simulink model "PWMGenerator"  (R2017a)
settings: Solver=VariableStepAuto  StartTime=0.0  StopTime=10.0  RelTol=1e-3
libraries: hdlsllib x15, simulink x5
settings Model: Creator=zhao.yi4  LastModifiedBy=zhao.yi4
settings OptimizationCC: BlockReduction=off  ConditionallyExecuteInputs=off  DefaultParameterBehavior=Inlined
settings DebuggingCC: AlgebraicLoopMsg=error
settings HardwareCC: ProdBitPerPointer=32  ProdBitPerSizeT=32  ProdBitPerPtrDiffT=32  ProdLargestAtomicFloat=None  ProdIntDivRoundTo=Undefined  ProdEndianess=Unspecified  ProdWordSize=32  ProdHWDeviceType=ASIC/FPGA->ASIC/FPGA  ProdEqTarget=off

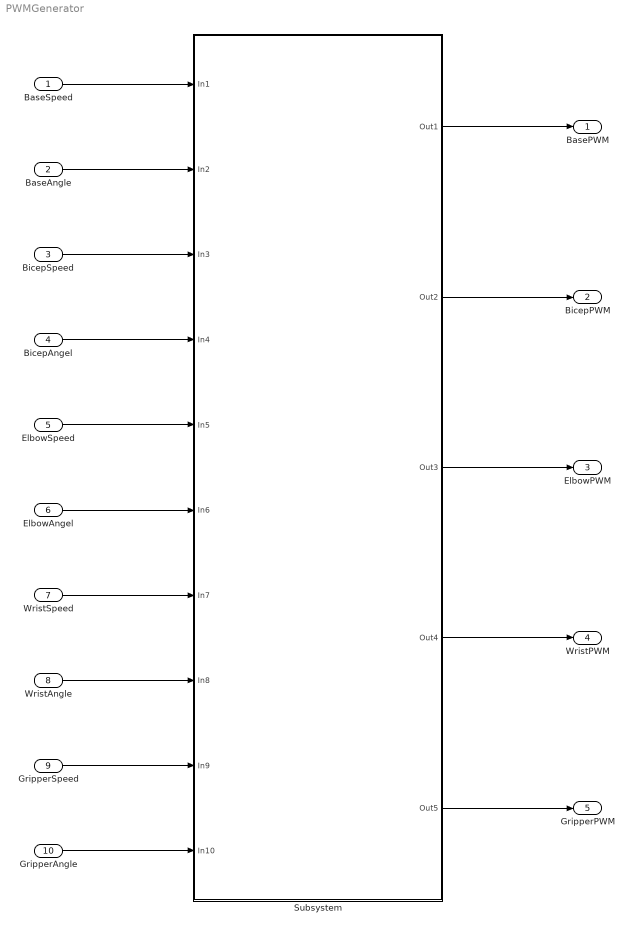
== system PWMGenerator ==
  BaseSpeed : Inport  OutDataTypeStr=uint8  SampleTime=1
  BaseAngle : Inport  Port=2  OutDataTypeStr=uint8  SampleTime=1
  BicepSpeed : Inport  Port=3  OutDataTypeStr=uint8  SampleTime=1
  BicepAngel : Inport  Port=4  OutDataTypeStr=uint8  SampleTime=1
  ElbowSpeed : Inport  Port=5  OutDataTypeStr=uint8  SampleTime=1
  ElbowAngel : Inport  Port=6  OutDataTypeStr=uint8  SampleTime=1
  WristSpeed : Inport  Port=7  OutDataTypeStr=uint8  SampleTime=1
  WristAngle : Inport  Port=8  OutDataTypeStr=uint8  SampleTime=1
  GripperSpeed : Inport  Port=9  OutDataTypeStr=uint8  SampleTime=1
  GripperAngle : Inport  Port=10  OutDataTypeStr=uint8  SampleTime=1
  Subsystem : Subsystem
  "BasePWM " : Outport  SampleTime=1
  "BicepPWM " : Outport  Port=2  SampleTime=1
  "ElbowPWM " : Outport  Port=3  SampleTime=1
  "WristPWM " : Outport  Port=4  SampleTime=1
  "GripperPWM " : Outport  Port=5  SampleTime=1
  wires:
  BaseSpeed/1 -> Subsystem/1(In1)
  BaseAngle/1 -> Subsystem/2(In2)
  BicepSpeed/1 -> Subsystem/3(In3)
  BicepAngel/1 -> Subsystem/4(In4)
  ElbowSpeed/1 -> Subsystem/5(In5)
  ElbowAngel/1 -> Subsystem/6(In6)
  WristSpeed/1 -> Subsystem/7(In7)
  WristAngle/1 -> Subsystem/8(In8)
  GripperSpeed/1 -> Subsystem/9(In9)
  GripperAngle/1 -> Subsystem/10(In10)
  Subsystem/1(Out1) -> "BasePWM "/1
  Subsystem/2(Out2) -> "BicepPWM "/1
  Subsystem/3(Out3) -> "ElbowPWM "/1
  Subsystem/4(Out4) -> "WristPWM "/1
  Subsystem/5(Out5) -> "GripperPWM "/1

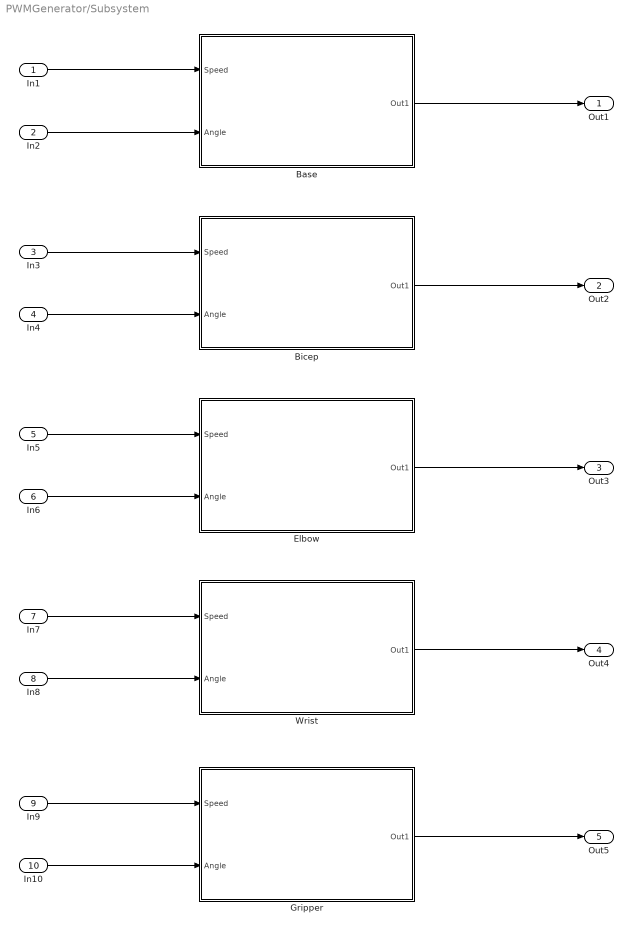
== system PWMGenerator/Subsystem ==
  In1 : Inport
  In2 : Inport  Port=2
  In3 : Inport  Port=3
  In4 : Inport  Port=4
  In5 : Inport  Port=5
  In6 : Inport  Port=6
  In7 : Inport  Port=7
  In8 : Inport  Port=8
  In9 : Inport  Port=9
  In10 : Inport  Port=10
  Base : Subsystem
  Bicep : Subsystem
  Elbow : Subsystem
  Gripper : Subsystem
  Wrist : Subsystem
  Out1 : Outport
  Out2 : Outport  Port=2
  Out3 : Outport  Port=3
  Out4 : Outport  Port=4
  Out5 : Outport  Port=5
  wires:
  Bicep/1(Out1) -> Out2/1
  In3/1 -> Bicep/1("Speed ")
  In4/1 -> Bicep/2(Angle)
  In1/1 -> Base/1("Speed ")
  In2/1 -> Base/2(Angle)
  Base/1(Out1) -> Out1/1
  In7/1 -> Wrist/1("Speed ")
  Wrist/1(Out1) -> Out4/1
  In8/1 -> Wrist/2(Angle)
  Elbow/1(Out1) -> Out3/1
  In6/1 -> Elbow/2(Angle)
  In5/1 -> Elbow/1("Speed ")
  Gripper/1(Out1) -> Out5/1
  In9/1 -> Gripper/1("Speed ")
  In10/1 -> Gripper/2(Angle)

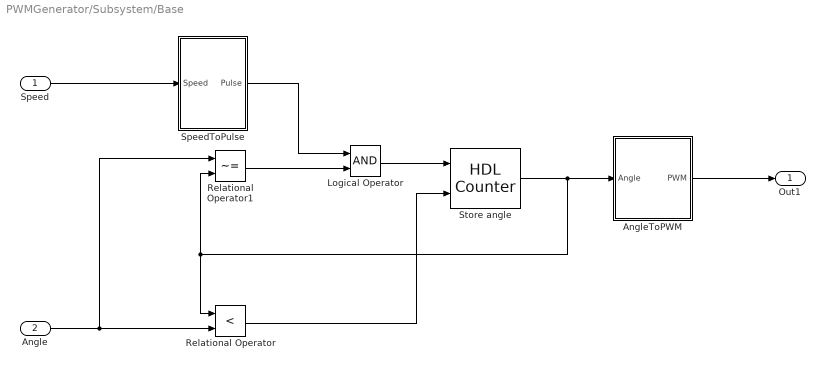
== system PWMGenerator/Subsystem/Base ==
  "Speed " : Inport  SampleTime=1
  Angle : Inport  Port=2  SampleTime=1
  "AngleToPWM " : Subsystem
  Logical Operator : Logic  AllPortsSameDT=off  OutDataTypeStr=boolean
  Relational Operator : RelationalOperator  Operator=<  OutDataTypeStr=boolean  RndMeth=Simplest
  Relational Operator1 : RelationalOperator  Operator=~=  OutDataTypeStr=boolean  RndMeth=Simplest
  SpeedToPulse : Subsystem
  Store angle : hdlsllib/HDL Operations/HDL Counter  CountType=Count limited  CountInit=90  CountStep=1  CountMax=185  CountFromType=Initial value  CountFrom=90  CountResetPort=off  CountLoadPort=off  CountEnbPort=on  CountDirPort=on  CountDataType=Unsigned  CountWordLen=8  CountFracLen=0  CountSampTime=1
      settings: SourceProductName=HDL Coder  SourceProductBaseCode=HD
  Out1 : Outport  SampleTime=1
  wires:
  "AngleToPWM "/1("PWM ") -> Out1/1
  Logical Operator/1 -> Store angle/1
  Store angle/1 -> Relational Operator1/2, Relational Operator/1, "AngleToPWM "/1(Angle)
  Relational Operator/1 -> Store angle/2
  Angle/1 -> Relational Operator1/1, Relational Operator/2
  SpeedToPulse/1("Pulse ") -> Logical Operator/1
  "Speed "/1 -> SpeedToPulse/1(Speed)
  Relational Operator1/1 -> Logical Operator/2

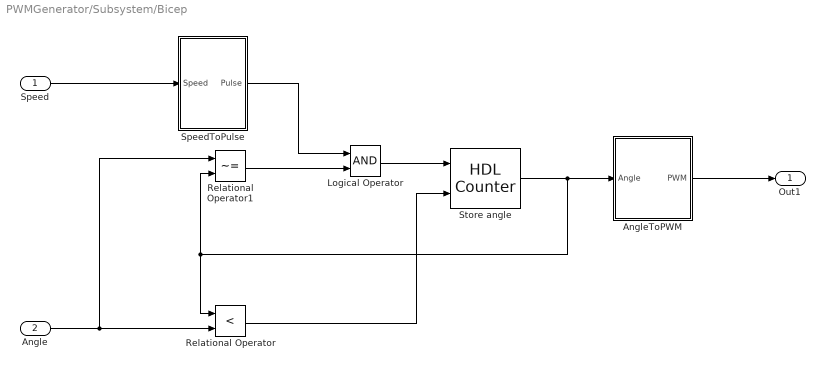
== system PWMGenerator/Subsystem/Bicep ==
  "Speed " : Inport  SampleTime=1
  Angle : Inport  Port=2  SampleTime=1
  "AngleToPWM " : Subsystem
  Logical Operator : Logic  AllPortsSameDT=off  OutDataTypeStr=boolean
  Relational Operator : RelationalOperator  Operator=<  OutDataTypeStr=boolean  RndMeth=Simplest
  Relational Operator1 : RelationalOperator  Operator=~=  OutDataTypeStr=boolean  RndMeth=Simplest
  SpeedToPulse : Subsystem
  Store angle : hdlsllib/HDL Operations/HDL Counter  CountType=Count limited  CountInit=90  CountStep=1  CountMax=185  CountFromType=Initial value  CountFrom=90  CountResetPort=off  CountLoadPort=off  CountEnbPort=on  CountDirPort=on  CountDataType=Unsigned  CountWordLen=8  CountFracLen=0  CountSampTime=1
      settings: SourceProductName=HDL Coder  SourceProductBaseCode=HD
  Out1 : Outport  SampleTime=1
  wires:
  "AngleToPWM "/1("PWM ") -> Out1/1
  Logical Operator/1 -> Store angle/1
  Store angle/1 -> Relational Operator1/2, Relational Operator/1, "AngleToPWM "/1(Angle)
  Relational Operator/1 -> Store angle/2
  Angle/1 -> Relational Operator1/1, Relational Operator/2
  SpeedToPulse/1("Pulse ") -> Logical Operator/1
  "Speed "/1 -> SpeedToPulse/1(Speed)
  Relational Operator1/1 -> Logical Operator/2

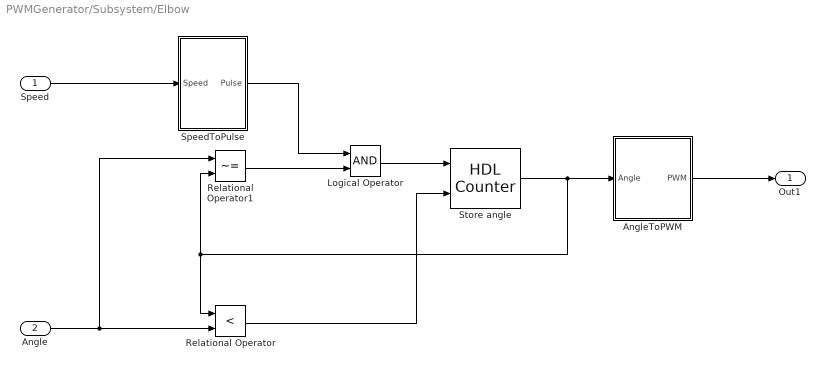
== system PWMGenerator/Subsystem/Elbow ==
  "Speed " : Inport  SampleTime=1
  Angle : Inport  Port=2  SampleTime=1
  "AngleToPWM " : Subsystem
  Logical Operator : Logic  AllPortsSameDT=off  OutDataTypeStr=boolean
  Relational Operator : RelationalOperator  Operator=<  OutDataTypeStr=boolean  RndMeth=Simplest
  Relational Operator1 : RelationalOperator  Operator=~=  OutDataTypeStr=boolean  RndMeth=Simplest
  SpeedToPulse : Subsystem
  Store angle : hdlsllib/HDL Operations/HDL Counter  CountType=Count limited  CountInit=90  CountStep=1  CountMax=185  CountFromType=Initial value  CountFrom=90  CountResetPort=off  CountLoadPort=off  CountEnbPort=on  CountDirPort=on  CountDataType=Unsigned  CountWordLen=8  CountFracLen=0  CountSampTime=1
      settings: SourceProductName=HDL Coder  SourceProductBaseCode=HD
  Out1 : Outport  SampleTime=1
  wires:
  "AngleToPWM "/1("PWM ") -> Out1/1
  Logical Operator/1 -> Store angle/1
  Store angle/1 -> Relational Operator1/2, Relational Operator/1, "AngleToPWM "/1(Angle)
  Relational Operator/1 -> Store angle/2
  Angle/1 -> Relational Operator1/1, Relational Operator/2
  SpeedToPulse/1("Pulse ") -> Logical Operator/1
  "Speed "/1 -> SpeedToPulse/1(Speed)
  Relational Operator1/1 -> Logical Operator/2

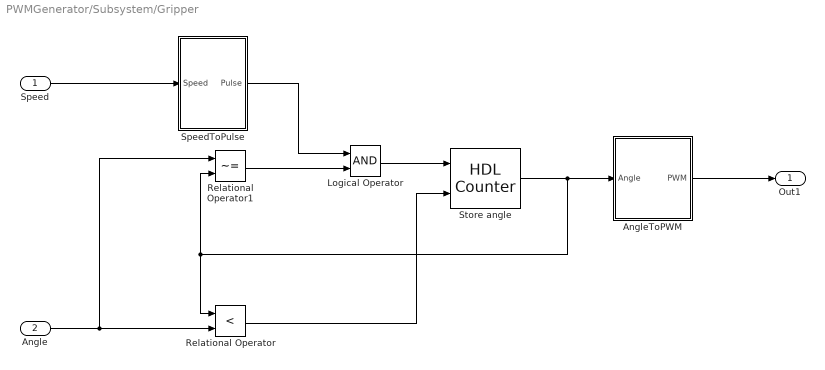
== system PWMGenerator/Subsystem/Gripper ==
  "Speed " : Inport  SampleTime=1
  Angle : Inport  Port=2  SampleTime=1
  "AngleToPWM " : Subsystem
  Logical Operator : Logic  AllPortsSameDT=off  OutDataTypeStr=boolean
  Relational Operator : RelationalOperator  Operator=<  OutDataTypeStr=boolean  RndMeth=Simplest
  Relational Operator1 : RelationalOperator  Operator=~=  OutDataTypeStr=boolean  RndMeth=Simplest
  SpeedToPulse : Subsystem
  Store angle : hdlsllib/HDL Operations/HDL Counter  CountType=Count limited  CountInit=90  CountStep=1  CountMax=185  CountFromType=Initial value  CountFrom=90  CountResetPort=off  CountLoadPort=off  CountEnbPort=on  CountDirPort=on  CountDataType=Unsigned  CountWordLen=8  CountFracLen=0  CountSampTime=1
      settings: SourceProductName=HDL Coder  SourceProductBaseCode=HD
  Out1 : Outport  SampleTime=1
  wires:
  "AngleToPWM "/1("PWM ") -> Out1/1
  Logical Operator/1 -> Store angle/1
  Store angle/1 -> Relational Operator1/2, Relational Operator/1, "AngleToPWM "/1(Angle)
  Relational Operator/1 -> Store angle/2
  Angle/1 -> Relational Operator1/1, Relational Operator/2
  SpeedToPulse/1("Pulse ") -> Logical Operator/1
  "Speed "/1 -> SpeedToPulse/1(Speed)
  Relational Operator1/1 -> Logical Operator/2

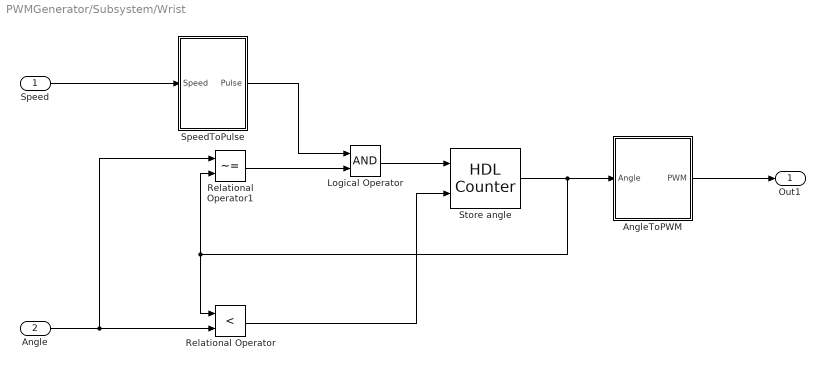
== system PWMGenerator/Subsystem/Wrist ==
  "Speed " : Inport  SampleTime=1
  Angle : Inport  Port=2  SampleTime=1
  "AngleToPWM " : Subsystem
  Logical Operator : Logic  AllPortsSameDT=off  OutDataTypeStr=boolean
  Relational Operator : RelationalOperator  Operator=<  OutDataTypeStr=boolean  RndMeth=Simplest
  Relational Operator1 : RelationalOperator  Operator=~=  OutDataTypeStr=boolean  RndMeth=Simplest
  SpeedToPulse : Subsystem
  Store angle : hdlsllib/HDL Operations/HDL Counter  CountType=Count limited  CountInit=90  CountStep=1  CountMax=185  CountFromType=Initial value  CountFrom=90  CountResetPort=off  CountLoadPort=off  CountEnbPort=on  CountDirPort=on  CountDataType=Unsigned  CountWordLen=8  CountFracLen=0  CountSampTime=1
      settings: SourceProductName=HDL Coder  SourceProductBaseCode=HD
  Out1 : Outport  SampleTime=1
  wires:
  "AngleToPWM "/1("PWM ") -> Out1/1
  Logical Operator/1 -> Store angle/1
  Store angle/1 -> Relational Operator1/2, Relational Operator/1, "AngleToPWM "/1(Angle)
  Relational Operator/1 -> Store angle/2
  Angle/1 -> Relational Operator1/1, Relational Operator/2
  SpeedToPulse/1("Pulse ") -> Logical Operator/1
  "Speed "/1 -> SpeedToPulse/1(Speed)
  Relational Operator1/1 -> Logical Operator/2

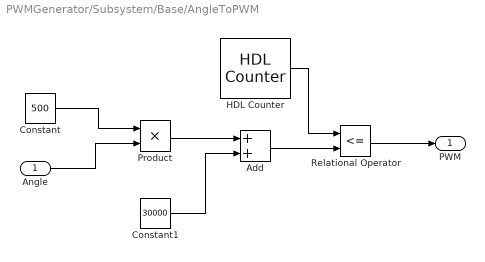
== system PWMGenerator/Subsystem/Base/AngleToPWM  ==
  Angle : Inport  OutDataTypeStr=uint8  SampleTime=1
  Add : Sum  AccumDataTypeStr=uint32  OutDataTypeStr=uint32
  Constant : Constant  Value=500  OutDataTypeStr=uint32  SampleTime=1
  Constant1 : Constant  Value=30000  OutDataTypeStr=uint32  SampleTime=1
  HDL Counter : hdlsllib/HDL Operations/HDL Counter  CountType=Count limited  CountInit=0  CountStep=1  CountMax=1000000  CountFromType=Initial value  CountFrom=0  CountResetPort=off  CountLoadPort=off  CountEnbPort=off  CountDirPort=off  CountDataType=Unsigned  CountWordLen=32  CountFracLen=0  CountSampTime=1
      settings: SourceProductName=HDL Coder  SourceProductBaseCode=HD
  Product : Product  OutDataTypeStr=uint32
  Relational Operator : RelationalOperator  Operator=<=  OutDataTypeStr=boolean  RndMeth=Simplest
  "PWM " : Outport  SampleTime=1
  wires:
  Product/1 -> Add/1
  Angle/1 -> Product/2
  Constant/1 -> Product/1
  HDL Counter/1 -> Relational Operator/1
  Relational Operator/1 -> "PWM "/1
  Add/1 -> Relational Operator/2
  Constant1/1 -> Add/2

== system PWMGenerator/Subsystem/Base/SpeedToPulse ==
  Speed : Inport  OutDataTypeStr=uint8  SampleTime=1
  Compare To Constant : simulink/Logic and Bit Operations/Compare To Constant  relop===  const=0  OutDataTypeStr=boolean
  Cycles in a second : Constant  Value=50000000  OutDataTypeStr=uint32  SampleTime=1
  Divide : Product  Inputs=*/  SaturateOnIntegerOverflow=on  RndMeth=Zero
  HDL Counter : hdlsllib/HDL Operations/HDL Counter  CountType=Free running  CountInit=0  CountStep=1  CountMax=25  CountFromType=Initial value  CountFrom=0  CountResetPort=on  CountLoadPort=off  CountEnbPort=off  CountDirPort=off  CountDataType=Unsigned  CountWordLen=32  CountFracLen=0  CountSampTime=1
      settings: SourceProductName=HDL Coder  SourceProductBaseCode=HD
  Relational Operator : RelationalOperator  Operator=>  OutDataTypeStr=boolean  RndMeth=Simplest
  "Pulse " : Outport  SampleTime=1
  wires:
  HDL Counter/1 -> Relational Operator/1, Compare To Constant/1
  Speed/1 -> Divide/2
  Relational Operator/1 -> HDL Counter/1
  Cycles in a second/1 -> Divide/1
  Divide/1 -> Relational Operator/2
  Compare To Constant/1 -> "Pulse "/1

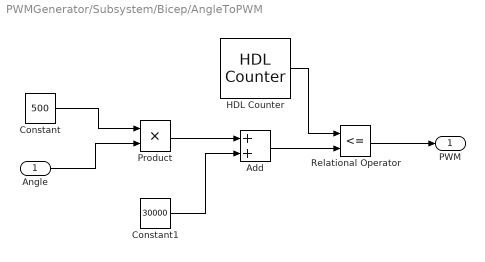
== system PWMGenerator/Subsystem/Bicep/AngleToPWM  ==
  Angle : Inport  OutDataTypeStr=uint8  SampleTime=1
  Add : Sum  AccumDataTypeStr=uint32  OutDataTypeStr=uint32
  Constant : Constant  Value=500  OutDataTypeStr=uint32  SampleTime=1
  Constant1 : Constant  Value=30000  OutDataTypeStr=uint32  SampleTime=1
  HDL Counter : hdlsllib/HDL Operations/HDL Counter  CountType=Count limited  CountInit=0  CountStep=1  CountMax=1000000  CountFromType=Initial value  CountFrom=0  CountResetPort=off  CountLoadPort=off  CountEnbPort=off  CountDirPort=off  CountDataType=Unsigned  CountWordLen=32  CountFracLen=0  CountSampTime=1
      settings: SourceProductName=HDL Coder  SourceProductBaseCode=HD
  Product : Product  OutDataTypeStr=uint32
  Relational Operator : RelationalOperator  Operator=<=  OutDataTypeStr=boolean  RndMeth=Simplest
  "PWM " : Outport  SampleTime=1
  wires:
  Product/1 -> Add/1
  Angle/1 -> Product/2
  Constant/1 -> Product/1
  HDL Counter/1 -> Relational Operator/1
  Relational Operator/1 -> "PWM "/1
  Add/1 -> Relational Operator/2
  Constant1/1 -> Add/2

== system PWMGenerator/Subsystem/Bicep/SpeedToPulse ==
  Speed : Inport  OutDataTypeStr=uint8  SampleTime=1
  Compare To Constant : simulink/Logic and Bit Operations/Compare To Constant  relop===  const=0  OutDataTypeStr=boolean
  Cycles in a second : Constant  Value=50000000  OutDataTypeStr=uint32  SampleTime=1
  Divide : Product  Inputs=*/  SaturateOnIntegerOverflow=on  RndMeth=Zero
  HDL Counter : hdlsllib/HDL Operations/HDL Counter  CountType=Free running  CountInit=0  CountStep=1  CountMax=25  CountFromType=Initial value  CountFrom=0  CountResetPort=on  CountLoadPort=off  CountEnbPort=off  CountDirPort=off  CountDataType=Unsigned  CountWordLen=32  CountFracLen=0  CountSampTime=1
      settings: SourceProductName=HDL Coder  SourceProductBaseCode=HD
  Relational Operator : RelationalOperator  Operator=>  OutDataTypeStr=boolean  RndMeth=Simplest
  "Pulse " : Outport  SampleTime=1
  wires:
  HDL Counter/1 -> Relational Operator/1, Compare To Constant/1
  Speed/1 -> Divide/2
  Relational Operator/1 -> HDL Counter/1
  Cycles in a second/1 -> Divide/1
  Divide/1 -> Relational Operator/2
  Compare To Constant/1 -> "Pulse "/1

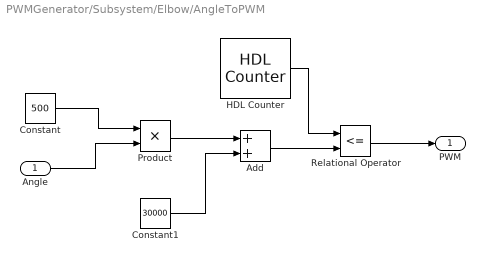
== system PWMGenerator/Subsystem/Elbow/AngleToPWM  ==
  Angle : Inport  OutDataTypeStr=uint8  SampleTime=1
  Add : Sum  AccumDataTypeStr=uint32  OutDataTypeStr=uint32
  Constant : Constant  Value=500  OutDataTypeStr=uint32  SampleTime=1
  Constant1 : Constant  Value=30000  OutDataTypeStr=uint32  SampleTime=1
  HDL Counter : hdlsllib/HDL Operations/HDL Counter  CountType=Count limited  CountInit=0  CountStep=1  CountMax=1000000  CountFromType=Initial value  CountFrom=0  CountResetPort=off  CountLoadPort=off  CountEnbPort=off  CountDirPort=off  CountDataType=Unsigned  CountWordLen=32  CountFracLen=0  CountSampTime=1
      settings: SourceProductName=HDL Coder  SourceProductBaseCode=HD
  Product : Product  OutDataTypeStr=uint32
  Relational Operator : RelationalOperator  Operator=<=  OutDataTypeStr=boolean  RndMeth=Simplest
  "PWM " : Outport  SampleTime=1
  wires:
  Product/1 -> Add/1
  Angle/1 -> Product/2
  Constant/1 -> Product/1
  HDL Counter/1 -> Relational Operator/1
  Relational Operator/1 -> "PWM "/1
  Add/1 -> Relational Operator/2
  Constant1/1 -> Add/2

== system PWMGenerator/Subsystem/Elbow/SpeedToPulse ==
  Speed : Inport  OutDataTypeStr=uint8  SampleTime=1
  Compare To Constant : simulink/Logic and Bit Operations/Compare To Constant  relop===  const=0  OutDataTypeStr=boolean
  Cycles in a second : Constant  Value=50000000  OutDataTypeStr=uint32  SampleTime=1
  Divide : Product  Inputs=*/  SaturateOnIntegerOverflow=on  RndMeth=Zero
  HDL Counter : hdlsllib/HDL Operations/HDL Counter  CountType=Free running  CountInit=0  CountStep=1  CountMax=25  CountFromType=Initial value  CountFrom=0  CountResetPort=on  CountLoadPort=off  CountEnbPort=off  CountDirPort=off  CountDataType=Unsigned  CountWordLen=32  CountFracLen=0  CountSampTime=1
      settings: SourceProductName=HDL Coder  SourceProductBaseCode=HD
  Relational Operator : RelationalOperator  Operator=>  OutDataTypeStr=boolean  RndMeth=Simplest
  "Pulse " : Outport  SampleTime=1
  wires:
  HDL Counter/1 -> Relational Operator/1, Compare To Constant/1
  Speed/1 -> Divide/2
  Relational Operator/1 -> HDL Counter/1
  Cycles in a second/1 -> Divide/1
  Divide/1 -> Relational Operator/2
  Compare To Constant/1 -> "Pulse "/1

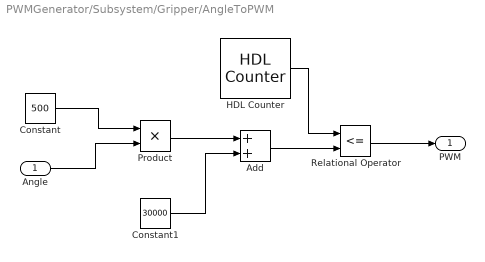
== system PWMGenerator/Subsystem/Gripper/AngleToPWM  ==
  Angle : Inport  OutDataTypeStr=uint8  SampleTime=1
  Add : Sum  AccumDataTypeStr=uint32  OutDataTypeStr=uint32
  Constant : Constant  Value=500  OutDataTypeStr=uint32  SampleTime=1
  Constant1 : Constant  Value=30000  OutDataTypeStr=uint32  SampleTime=1
  HDL Counter : hdlsllib/HDL Operations/HDL Counter  CountType=Count limited  CountInit=0  CountStep=1  CountMax=1000000  CountFromType=Initial value  CountFrom=0  CountResetPort=off  CountLoadPort=off  CountEnbPort=off  CountDirPort=off  CountDataType=Unsigned  CountWordLen=32  CountFracLen=0  CountSampTime=1
      settings: SourceProductName=HDL Coder  SourceProductBaseCode=HD
  Product : Product  OutDataTypeStr=uint32
  Relational Operator : RelationalOperator  Operator=<=  OutDataTypeStr=boolean  RndMeth=Simplest
  "PWM " : Outport  SampleTime=1
  wires:
  Product/1 -> Add/1
  Angle/1 -> Product/2
  Constant/1 -> Product/1
  HDL Counter/1 -> Relational Operator/1
  Relational Operator/1 -> "PWM "/1
  Add/1 -> Relational Operator/2
  Constant1/1 -> Add/2

== system PWMGenerator/Subsystem/Gripper/SpeedToPulse ==
  Speed : Inport  OutDataTypeStr=uint8  SampleTime=1
  Compare To Constant : simulink/Logic and Bit Operations/Compare To Constant  relop===  const=0  OutDataTypeStr=boolean
  Cycles in a second : Constant  Value=50000000  OutDataTypeStr=uint32  SampleTime=1
  Divide : Product  Inputs=*/  SaturateOnIntegerOverflow=on  RndMeth=Zero
  HDL Counter : hdlsllib/HDL Operations/HDL Counter  CountType=Free running  CountInit=0  CountStep=1  CountMax=25  CountFromType=Initial value  CountFrom=0  CountResetPort=on  CountLoadPort=off  CountEnbPort=off  CountDirPort=off  CountDataType=Unsigned  CountWordLen=32  CountFracLen=0  CountSampTime=1
      settings: SourceProductName=HDL Coder  SourceProductBaseCode=HD
  Relational Operator : RelationalOperator  Operator=>  OutDataTypeStr=boolean  RndMeth=Simplest
  "Pulse " : Outport  SampleTime=1
  wires:
  HDL Counter/1 -> Relational Operator/1, Compare To Constant/1
  Speed/1 -> Divide/2
  Relational Operator/1 -> HDL Counter/1
  Cycles in a second/1 -> Divide/1
  Divide/1 -> Relational Operator/2
  Compare To Constant/1 -> "Pulse "/1

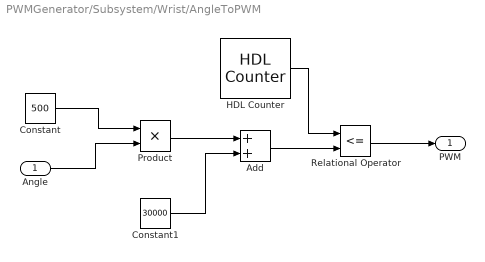
== system PWMGenerator/Subsystem/Wrist/AngleToPWM  ==
  Angle : Inport  OutDataTypeStr=uint8  SampleTime=1
  Add : Sum  AccumDataTypeStr=uint32  OutDataTypeStr=uint32
  Constant : Constant  Value=500  OutDataTypeStr=uint32  SampleTime=1
  Constant1 : Constant  Value=30000  OutDataTypeStr=uint32  SampleTime=1
  HDL Counter : hdlsllib/HDL Operations/HDL Counter  CountType=Count limited  CountInit=0  CountStep=1  CountMax=1000000  CountFromType=Initial value  CountFrom=0  CountResetPort=off  CountLoadPort=off  CountEnbPort=off  CountDirPort=off  CountDataType=Unsigned  CountWordLen=32  CountFracLen=0  CountSampTime=1
      settings: SourceProductName=HDL Coder  SourceProductBaseCode=HD
  Product : Product  OutDataTypeStr=uint32
  Relational Operator : RelationalOperator  Operator=<=  OutDataTypeStr=boolean  RndMeth=Simplest
  "PWM " : Outport  SampleTime=1
  wires:
  Product/1 -> Add/1
  Angle/1 -> Product/2
  Constant/1 -> Product/1
  HDL Counter/1 -> Relational Operator/1
  Relational Operator/1 -> "PWM "/1
  Add/1 -> Relational Operator/2
  Constant1/1 -> Add/2

== system PWMGenerator/Subsystem/Wrist/SpeedToPulse ==
  Speed : Inport  OutDataTypeStr=uint8  SampleTime=1
  Compare To Constant : simulink/Logic and Bit Operations/Compare To Constant  relop===  const=0  OutDataTypeStr=boolean
  Cycles in a second : Constant  Value=50000000  OutDataTypeStr=uint32  SampleTime=1
  Divide : Product  Inputs=*/  SaturateOnIntegerOverflow=on  RndMeth=Zero
  HDL Counter : hdlsllib/HDL Operations/HDL Counter  CountType=Free running  CountInit=0  CountStep=1  CountMax=25  CountFromType=Initial value  CountFrom=0  CountResetPort=on  CountLoadPort=off  CountEnbPort=off  CountDirPort=off  CountDataType=Unsigned  CountWordLen=32  CountFracLen=0  CountSampTime=1
      settings: SourceProductName=HDL Coder  SourceProductBaseCode=HD
  Relational Operator : RelationalOperator  Operator=>  OutDataTypeStr=boolean  RndMeth=Simplest
  "Pulse " : Outport  SampleTime=1
  wires:
  HDL Counter/1 -> Relational Operator/1, Compare To Constant/1
  Speed/1 -> Divide/2
  Relational Operator/1 -> HDL Counter/1
  Cycles in a second/1 -> Divide/1
  Divide/1 -> Relational Operator/2
  Compare To Constant/1 -> "Pulse "/1
